simulink model "mdl_GPSreceiveBin1_monitor"  (R2020b)
settings: Solver=FixedStepDiscrete  StartTime=0.0  StopTime=inf  RelTol=1e-3  EnableMultiTasking=on
undefined symbols (not defined in the file): Green, led0
libraries: simulink x1, raspberrypiBasiclib x1, raspberrypiCommlib x1
settings Model: ModifiedByFormat=The MathWorks Inc.  SimulationMode=external  EnablePacing=on  Creator=The MathWorks, Inc.  LastModifiedBy=The MathWorks Inc.
settings SolverCC: PositivePriorityOrder=on
settings DataIOCC: LimitDataPoints=on  SaveFormat=Array  ReturnWorkspaceOutputs=off
settings OptimizationCC: LifeSpan=1  MaxStackSize=64
settings DebuggingCC: UnderspecifiedInitializationDetection=Classic  MergeDetectMultiDrivingBlocksExec=none  SolverPrmCheckMsg=warning  AllowSymbolicDim=off  SFUnexpectedBacktrackingDiag=warning  SFNoUnconditionalDefaultTransitionDiag=warning  SFExecutionAtInitializationDiag=none  ArithmeticOperatorsInVariantConditions=warning
settings HardwareCC: ProdBitPerPointer=32  ProdBitPerSizeT=32  ProdBitPerPtrDiffT=32  ProdLargestAtomicInteger=Long  ProdLargestAtomicFloat=Double  ProdWordSize=32  ProdHWDeviceType=ARM Compatible->ARM Cortex  UseEmbeddedCoderFeatures=off  UseSimulinkCoderFeatures=off
settings ModelReferenceCC: PropagateSignalLabelsOutOfModel=off
settings SFSimCC: SimUseLocalCustomCode=off  MATLABDynamicMemAlloc=off  CustomCodeUndefinedFunction=UseInterfaceOnly
settings RTWCC: Description=Embedded Coder  SystemTargetFile=ert.tlc  HardwareBoard=Raspberry Pi  TemplateMakefile=ert_default_tmf  RTWUseLocalCustomCode=off  Toolchain=GNU GCC Raspberry Pi
settings CodeAppCC: MangleLength=10  StateflowObjectComments=on
settings ERTTargetCC: MultiwordLength=2048  ERTCustomFileBanners=off  SupportContinuousTime=on  SupportNonInlinedSFcns=on  RemoveResetFunc=off  ModelStepFunctionPrototypeControlCompliant=off  ConvertIfToSwitch=off  SuppressUnreachableDefaultCases=off
settings ConfigComp: CovMetricSettings=dw  CovSaveCumulativeToWorkspaceVar=on  CovSaveSingleToWorkspaceVar=on  CovExternalEMLEnable=off  CovSFcnEnable=off

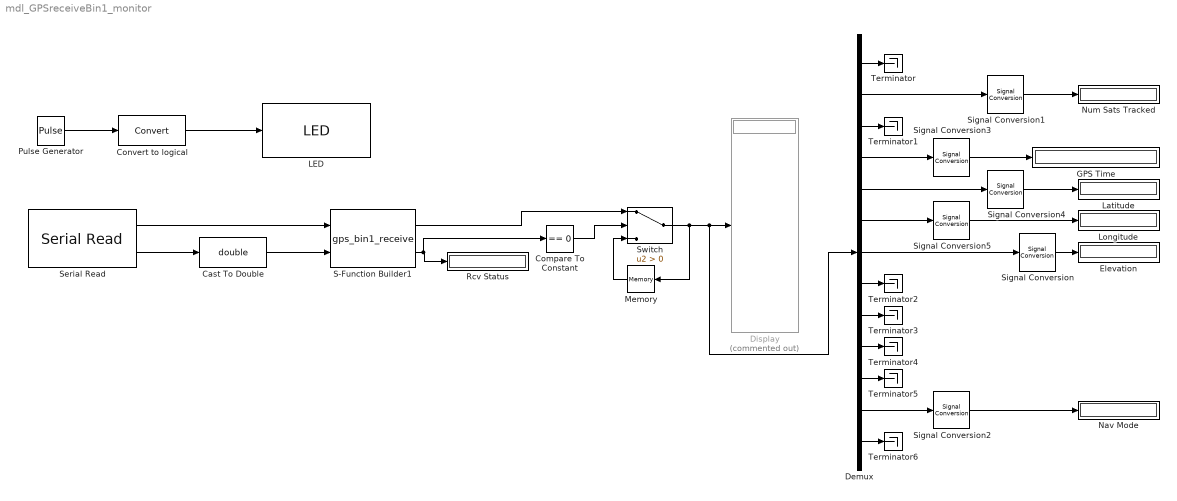
== system mdl_GPSreceiveBin1_monitor ==
  Cast To Double : DataTypeConversion  OutDataTypeStr=double
  Compare To Constant : simulink/Logic and Bit Operations/Compare To Constant  relop===  const=0  OutDataTypeStr=uint8
  Convert to logical : DataTypeConversion
  Demux : Demux  Outputs=13
  Display : Display  Commented=on
  Elevation : Display
  GPS Time : Display
      settings: Format=long_e
  LED : raspberrypiBasiclib/LED  BoardProperty=Pi 4 Model B  LED_=led0 (Green)
      settings: SourceProductName=Simulink Support Package for Raspberry Pi Hardware
  Latitude : Display
  Longitude : Display
  Memory : Memory
  Nav Mode : Display
  Num Sats Tracked : Display
  Pulse Generator : DiscretePulseGenerator  Period=10  PulseWidth=5  SampleTime=0.1
  Rcv Status : Display
  S-Function Builder1 : S-Function  FunctionName=gps_bin1_receive  SFunctionModules=gps_bin1_receive_wrapper  SFunctionDeploymentMode=off  EnableBusSupport=off  mask(S-Function Builder){}
      mask help: Simulink:masks:SFunctionBuilder_MD
      mask init:
      | val = [[.9  0.75 0.75 1 1 .9 .9 1]',[1 1 0.75 0.75 .9 .9 1 .9]'];try , sys = get_param(gcb,'SfunBuilderFcnName');if isempty(sys), sys = get_param(gcb,'FunctionName'); end,catch, sys = get_param(gcb,'FunctionName'); end
      settings: CopyFcn=set_param(gcbh,'LinkStatus','none')  OpenFcn=sfunctionwizard(gcbh)
      mask Display: plot(val(:,1),val(:,2)),disp(sys),port_label('input',1,'u0'),port_label('input',2,'u1'),port_label('output',1,'y0'),port_label('output',2,'y1')
  Serial Read : raspberrypiCommlib/Serial Read  board=Pi 4 Model B  SCIModule_=/dev/serial0  Baudrate_=19200  Parity=None  StopBits_=1  HardwareFlowControl=None  ByteOrder=LittleEndian  DataLength=64  DataType=uint8  OutputStatus=on  SampleTime=0.02  blockPlatform=RaspberryPi
      settings: SourceProductBaseCode=RASPPI
  Signal Conversion{,1..5} (6 alike) : SignalConversion  OverrideOpt=off
  Switch : Switch  Criteria=u2 > Threshold
  Terminator{,1..6} (7 alike) : Terminator
  wires:
  Pulse Generator/1 -> Convert to logical/1
  Convert to logical/1 -> LED/1
  Serial Read/1 -> S-Function Builder1/1
  S-Function Builder1/2 -> Compare To Constant/1, Rcv Status/1
  Serial Read/2 -> Cast To Double/1
  Cast To Double/1 -> S-Function Builder1/2
  Demux/2 -> Signal Conversion1/1
  Demux/5 -> Signal Conversion4/1
  Demux/6 -> Signal Conversion5/1
  Demux/7 -> Signal Conversion/1
  Demux/4 -> Signal Conversion3/1
  Demux/1 -> Terminator/1
  Demux/3 -> Terminator1/1
  Demux/8 -> Terminator2/1
  Demux/9 -> Terminator3/1
  Demux/10 -> Terminator4/1
  Demux/11 -> Terminator5/1
  Demux/12 -> Signal Conversion2/1
  Demux/13 -> Terminator6/1
  Signal Conversion/1 -> Elevation/1
  Signal Conversion1/1 -> Num Sats Tracked/1
  Signal Conversion3/1 -> GPS Time/1
  Signal Conversion4/1 -> Latitude/1
  Signal Conversion5/1 -> Longitude/1
  S-Function Builder1/1 -> Switch/1
  Switch/1 -> Memory/1, Demux/1, Display/1
  Memory/1 -> Switch/3
  Compare To Constant/1 -> Switch/2
  Signal Conversion2/1 -> Nav Mode/1
